simulink model "Feedback_Configuration_1"  (R2024b)
settings: Solver=VariableStepAuto  StartTime=0.0  StopTime=10.0  RelTol=1e-3
undefined symbols (not defined in the file or in its folder): k, r
libraries: cstblocks x3
settings Model: Creator=wilbe  LastModifiedBy=wilbe

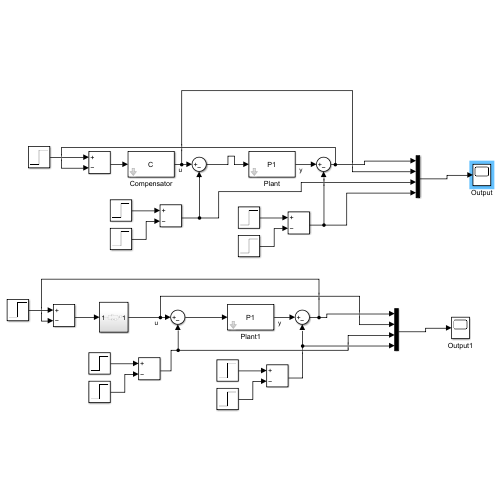
[thumbnail: Simulink's stored preview of the top-level diagram]
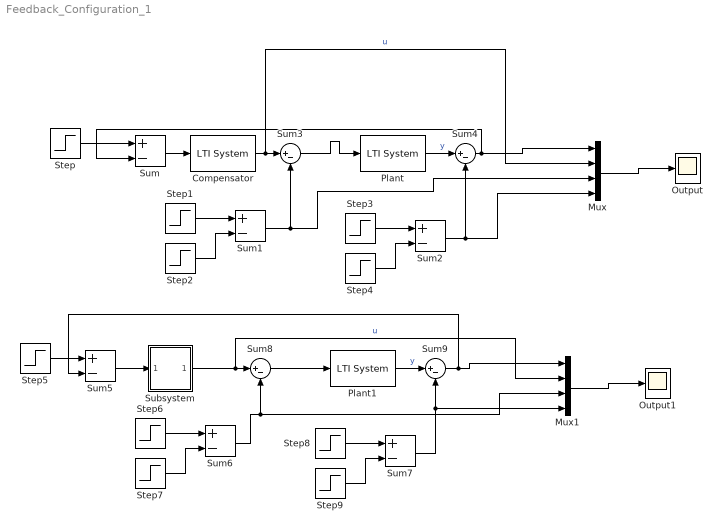
== system Feedback_Configuration_1 ==
  Compensator : cstblocks/LTI System  sys=C  IC=[]  PadeOrder=0
  Mux : Mux
  Mux1 : Mux
  Output : Scope
  Output1 : Scope
  Plant : cstblocks/LTI System  sys=P1  IC=[]  PadeOrder=0
  Plant1 : cstblocks/LTI System  sys=P1  IC=[]  PadeOrder=0
  Step : Step  Time=0  After=4  SampleTime=0
  Step1 : Step  Time=2  After=0.5  SampleTime=0
  Step2 : Step  Time=3  After=0.5  SampleTime=0
  Step3 : Step  Time=5  After=0.5  SampleTime=0
  Step4 : Step  Time=7  After=0.5  SampleTime=0
  Step5 : Step  Time=0  After=4  SampleTime=0
  Step6 : Step  Time=2  After=0.5  SampleTime=0
  Step7 : Step  Time=3  After=0.5  SampleTime=0
  Step8 : Step  Time=5  After=0.5  SampleTime=0
  Step9 : Step  Time=7  After=0.5  SampleTime=0
  Subsystem : Subsystem
  Sum{,1..2,5..7} (6 alike) : Sum  Inputs=+-
  Sum{3..4,8..9} (4 alike) : Sum  Inputs=|+-
  wires:
  Sum/1 -> Compensator/1
  Step/1 -> Sum/1
  Step1/1 -> Sum1/1
  Step2/1 -> Sum1/2
  Step4/1 -> Sum2/2
  Step3/1 -> Sum2/1
  Sum2/1 -> Mux/4, Sum4/2
  Compensator/1 -> Mux/2, Sum3/1  "u"
  Sum1/1 -> Mux/3, Sum3/2
  Sum3/1 -> Plant/1
  Plant/1 -> Sum4/1  "y"
  Sum4/1 -> Sum/2, Mux/1
  Mux/1 -> Output/1
  Subsystem/1(Out1) -> Mux1/2, Sum8/1  "u"
  Sum7/1 -> Mux1/4, Sum9/2
  Step7/1 -> Sum6/2
  Sum8/1 -> Plant1/1
  Sum9/1 -> Sum5/2, Mux1/1
  Step8/1 -> Sum7/1
  Step6/1 -> Sum6/1
  Plant1/1 -> Sum9/1  "y"
  Step9/1 -> Sum7/2
  Sum6/1 -> Mux1/3, Sum8/2
  Mux1/1 -> Output1/1
  Step5/1 -> Sum5/1
  Sum5/1 -> Subsystem/1(In1)

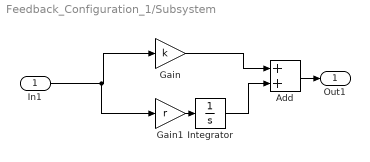
== system Feedback_Configuration_1/Subsystem ==
  In1 : Inport
  Add : Sum
  Gain : Gain  Gain=k
  Gain1 : Gain  Gain=r
  Integrator : Integrator
  Out1 : Outport
  wires:
  Gain1/1 -> Integrator/1
  In1/1 -> Gain1/1, Gain/1
  Integrator/1 -> Add/2
  Gain/1 -> Add/1
  Add/1 -> Out1/1
